simulink model "PendulumCart_Block"  (R2023a)
settings: Solver=ode45  StartTime=0.0  StopTime=3  RelTol=1e-3  EnableMultiTasking=on
values from neighbouring files (symbols this model uses):
  CG = -1.0944    [PendulumCart_Parameters_Mids.m]
  g = 9.81    [PendulumCart_Parameters_Mids.m]
  K = [-1.4584 -9.0946 -1.1371 -1.0944]    [PendulumCart_Parameters_Mids.m]
  l = 0.337    [PendulumCart_Parameters_Mids.m]
  m = 0.125    [PendulumCart_Parameters_Mids.m]
  M = 0.261    [PendulumCart_Parameters_Mids.m]
  r = 0.1    [PendulumCart_Parameters_Mids.m]
  theta_0 = 0.0    (= 0)    [PendulumCart_Parameters_Mids.m]
  theta_dot_0 = 0.0    (= 0)    [PendulumCart_Parameters_Mids.m]
  x_0 = 0.0    (= 0)    [PendulumCart_Parameters_Mids.m]
  x_dot_0 = 0.0    (= 0)    [PendulumCart_Parameters_Mids.m]
settings Model: Creator=rodrigue  LastModifiedBy=m260477
settings SolverCC: AlgebraicLoopSolver=TrustRegion
settings DataIOCC: LimitDataPoints=on  SaveFormat=Array  ReturnWorkspaceOutputs=off
settings OptimizationCC: LifeSpan=inf
settings DebuggingCC: UnderspecifiedInitializationDetection=Classic  MergeDetectMultiDrivingBlocksExec=none  SolverPrmCheckMsg=warning  UnconnectedInputMsg=warning  UnconnectedOutputMsg=warning  UnconnectedLineMsg=warning  StateNameClashWarn=warning  SFUnexpectedBacktrackingDiag=warning  SFNoUnconditionalDefaultTransitionDiag=warning  SFExecutionAtInitializationDiag=none  ArithmeticOperatorsInVariantConditions=warning
settings HardwareCC: ProdBitPerPointer=32  ProdBitPerSizeT=32  ProdBitPerPtrDiffT=32  ProdLargestAtomicFloat=None  ProdIntDivRoundTo=Undefined  ProdEndianess=Unspecified  ProdWordSize=32  ProdHWDeviceType=32-bit Generic
settings ModelReferenceCC: EnableRefExpFcnMdlSchedulingChecks=on  PropagateSignalLabelsOutOfModel=off
settings SFSimCC: SimUseLocalCustomCode=off  CustomCodeUndefinedFunction=UseInterfaceOnly
settings RTWCC: RTWUseLocalCustomCode=off
settings CodeAppCC: StateflowObjectComments=on
settings GRTTargetCC: TargetLangStandard=C89/C90 (ANSI)
settings ConfigComp: CovMetricSettings=dw  CovSaveCumulativeToWorkspaceVar=on  CovSaveSingleToWorkspaceVar=on  CovExternalEMLEnable=off

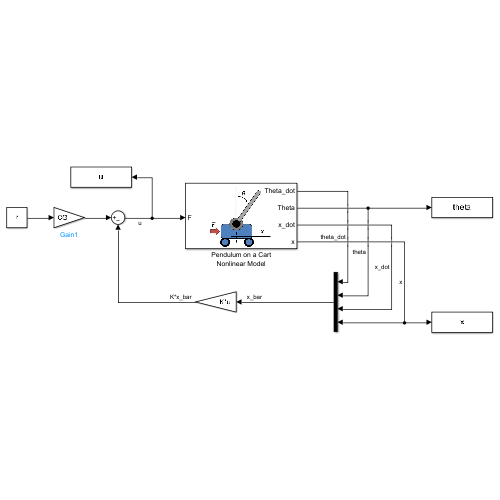
[thumbnail: Simulink's stored preview of the top-level diagram]
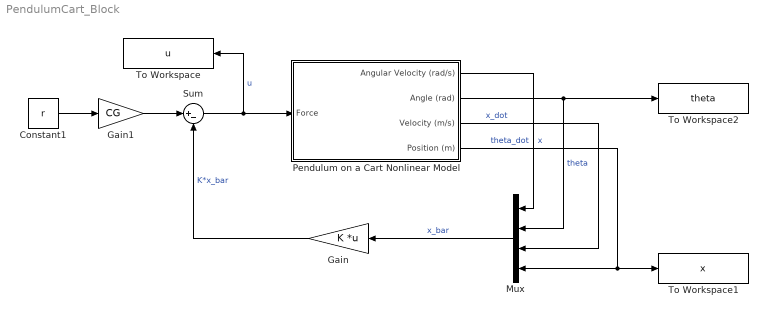
== system PendulumCart_Block ==
  Constant1 : Constant  Value=r
  Gain : Gain  Gain=K  Multiplication=Matrix(K*u)
  Gain1 : Gain  Gain=CG
  Mux : Mux
  Pendulum on a Cart Nonlinear Model : Subsystem  Description=Nonlinear of the Pendulum on a Cart. The input is the horizontal force applied to the cart.
      mask Display:
      | image('PendulumCartImage.jpg')
      | port_label('input', 1, 'F')
      | port_label('output', 1, 'Theta_dot')
      | port_label('output', 2, 'Theta')
      | port_label('output', 3, 'x_dot')
      | port_label('output', 4, 'x')
  Sum : Sum  Inputs=|+-
  To Workspace : ToWorkspace  VariableName=u  SampleTime=-1
  To Workspace1 : ToWorkspace  VariableName=x  SampleTime=-1
  To Workspace2 : ToWorkspace  VariableName=theta  SampleTime=-1
  wires:
  Mux/1 -> Gain/1  "x_bar"
  Sum/1 -> To Workspace/1, Pendulum on a Cart Nonlinear Model/1(Force)  "u"
  Pendulum on a Cart Nonlinear Model/1(Angular Velocity (rad/s)) -> Mux/1  "theta_dot"
  Pendulum on a Cart Nonlinear Model/2(Angle (rad)) -> To Workspace2/1, Mux/2  "theta"
  Pendulum on a Cart Nonlinear Model/3(Velocity (m/s)) -> Mux/3  "x_dot"
  Pendulum on a Cart Nonlinear Model/4(Position (m)) -> To Workspace1/1, Mux/4  "x"
  Gain/1 -> Sum/2  "K*x_bar"
  Constant1/1 -> Gain1/1
  Gain1/1 -> Sum/1

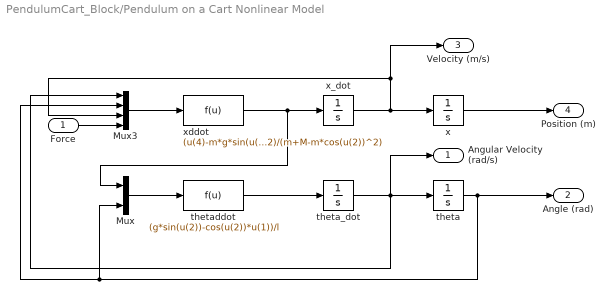
== system PendulumCart_Block/Pendulum on a Cart Nonlinear Model ==
  Force : Inport
  Mux : Mux  Inputs=2
  Mux3 : Mux
  theta : Integrator  InitialCondition=theta_0  ContinuousStateAttributes='theta'
  theta_dot : Integrator  InitialCondition=theta_dot_0  ContinuousStateAttributes='thetadot'
  thetaddot : Fcn  Expr=(g*sin(u(2))-cos(u(2))*u(1))/l
  x : Integrator  InitialCondition=x_0  ContinuousStateAttributes='x'
  x_dot : Integrator  InitialCondition=x_dot_0  ContinuousStateAttributes='xdot'
  xddot : Fcn  Expr=(u(4)-m*g*sin(u(2))*cos(u(2))+m*l*sin(u(2))*u(1)^2)/(m+M-m*cos(u(2))^2)
  Angular Velocity (rad/s) : Outport
  Angle (rad) : Outport  Port=2
  Velocity (m/s) : Outport  Port=3
  Position (m) : Outport  Port=4
  wires:
  Mux3/1 -> xddot/1
  theta_dot/1 -> Angular Velocity (rad/s)/1, theta/1, Mux3/1
  Force/1 -> Mux3/4
  x_dot/1 -> Velocity (m/s)/1, Mux3/3, x/1
  Mux/1 -> thetaddot/1
  xddot/1 -> Mux/1, x_dot/1
  thetaddot/1 -> theta_dot/1
  theta/1 -> Mux/2, Mux3/2, Angle (rad)/1
  x/1 -> Position (m)/1
